simulink model "water_4hopper_open"  (Simulink 8.0)
settings: Solver=ode23  StartTime=0.0  StopTime=30  RelTol=1e-4
values from neighbouring files (symbols this model uses):
  alpha = 30    [SimParam_4VDF.m]
  C_d = 0.703    [SimParam_4VDF.m]
  density = 1000    [SimParam_4VDF.m]
  dTorqueAmp = 0    [SimParam_4VDF.m]
  dTorqueFreq = 0.5    [SimParam_4VDF.m]
  dTorquePhase = 2*pi*rand(1,4)    [SimParam_4VDF.m]
  frame_inertia = diag([Ix,Iy,Iz])    [SimParam_4VDF.m]
  freq = 60    [SimParam_4VDF.m]
  g = 9.81    [SimParam_4VDF.m]
  leg_length = 0.0249    [SimParam_4VDF.m]
  mass = 0.1    [SimParam_4VDF.m]
  S1 = pi*r1^2*0.9185    (= 0.00115422114093)    [SimParam_4VDF.m]
  S2 = pi*r2^2*0.9185    (= 7.21388213081e-05)    [SimParam_4VDF.m]
  tau = 0.005    [SimParam_4VDF.m]
  waveAmp = 0    [SimParam_4VDF.m]
  waveFreq = 0.5    [SimParam_4VDF.m]
undefined symbols (not defined in the file): amp, cw_FL_HL, cw_FR_FL, cw_FR_HR, cw_HR_HL, FL_HL_lag, FR_FL_lag, FR_HR_lag, HR_HL_lag, wavePhase, y_0
libraries: mblibv1 x33
(part 1 of 2)
settings Model: Creator=Metti  LastModifiedBy=nitisht  SimulationMode=rapid-accelerator
settings SolverCC: ZeroCrossControl=DisableAll
settings DataIOCC: SignalLoggingSaveFormat=ModelDataLogs
settings DebuggingCC: FcnCallInpInsideContextMsg=EnableAllAsWarning
settings SimMechanicsCC: VisSampleTime=0.05  AutoFitVis=GROWTOFIT  LastVizWinPosition=[1 41 1600 759]  CamPosition=[-6.20117;3.01965;9.86212;]  CamTarget=[-0.265896;0.0450483;0.16365;]  CamUpVector=[0.0887544;0.966202;-0.242026;]  CamHeight=0.984746  VisBackgroundColor=[0.9;0.9;0.95;]  DefaultBodyColor=[1;0;0;]
settings ConfigurationSet: Description=SimMechanics 2G

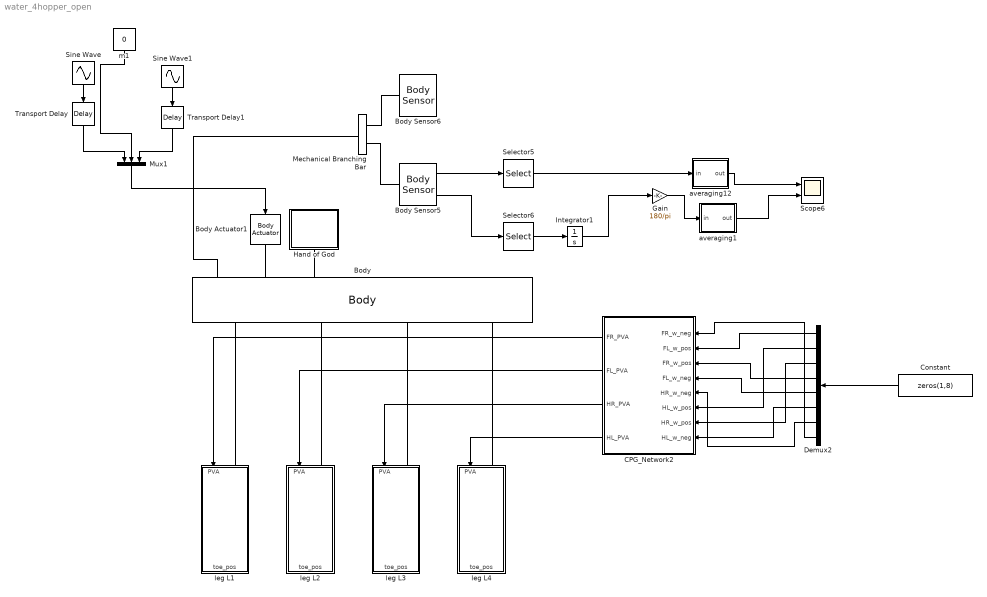
== system water_4hopper_open ==
  Body : mblibv1/Bodies/Body  LConnTagsString=CG|CS10|CS1|CS6|CS7|CS8|CS9  RConnTagsString=CS2|CS3|CS4|CS5  UpdateFromCAD=off  DialogClass=MechanicalBodyBlock  Mass=mass  MassUnits=kg  InertiaUnits=kg*m^2  Inertia=frame_inertia  Shape=Cylinder  ShapeDims=[1 1]  ShapeUnits=m  ShapeUse=false  Density=1  DensityUnits=kg/m^3  DensityUse=false  GraphicsMode=MACHINE_DEFAULT  BodyColorSelMode=MACHINE_DEFAULT  BodyColor=[1 0 0]  AttachedToCS=CG  CG=Left$CG$CG_pos$CS1$CS1$m$[0 0 0]$Euler X-Y-Z$deg$WORLD$true$none  WorkingFrames=Left$CS10$CG_pos$CS1$CS1$m$[0 0 0]$Euler X-Y-Z$deg$WORLD$true$none#Left$CS1$[0 0 0]$Adjoining$Adjoining$m$[0 0 0]$Euler X-Y-Z$deg$WORLD$true$none#Right$CS2$TR_FR$CS1$CS1$m$[0 0 0]$Euler X-Y-Z$deg$WORLD$true$none#Left$CS6$TR_FR$CS1$CS1$m$[0 0 0]$Euler X-Y-Z$deg$WORLD$true$none#Right$CS3$TR_FL$CS1$CS1$m$[0 0 0]$Euler X-Y-Z$deg$WORLD$true$none#Left$CS7$TR_FL$CS1$CS1$m$[0 0 0]$Euler X-Y-Z$deg$WORLD$true$none#Right$CS4$TR_HR$CS1$CS1$m$[0 0 0]$Euler X-Y-Z$deg$WORLD$true$none#Left$CS8$TR_HR$CS1$CS1$m$[0 0 0]$Euler X-Y-Z$deg$WORLD$true$none#Right$CS5$TR_HL$CS1$CS1$m$[0 0 0]$Euler X-Y-Z$deg$WORLD$true$none#Left$CS9$TR_HL$CS1$CS1$m$[0 0 0]$Euler X-Y-Z$deg$WORLD$true$none  CGPos=CG_pos  CGRot=[0 0 0]  CS0Pos=[]  CS0Rot=[]  CS1Pos=[0 0 0]  CS1Rot=[0 0 0]  CS2Pos=TR_FR  CS2Rot=[0 0 0]  CS3Pos=TR_FL  CS3Rot=[0 0 0]  CS4Pos=TR_HR  CS4Rot=[0 0 0]  CS5Pos=TR_HL  CS5Rot=[0 0 0]  CS6Pos=TR_FR  CS6Rot=[0 0 0]  CS7Pos=TR_FL  CS7Rot=[0 0 0]  CS8Pos=TR_HR  CS8Rot=[0 0 0]  CS9Pos=TR_HL  CS9Rot=[0 0 0]  CS10Pos=CG_pos  CS10Rot=[0 0 0]  CS11Pos=[]  CS11Rot=[]  CS12Pos=[]  CS12Rot=[]  CS13Pos=[]  CS13Rot=[]  CS14Pos=[]  CS14Rot=[]  CS15Pos=[]  CS15Rot=[]  CS16Pos=[]  CS16Rot=[]  CS17Pos=[]  CS17Rot=[]  CS18Pos=[]  CS18Rot=[]  CS19Pos=[]  CS19Rot=[]  CS20Pos=[]  CS20Rot=[]
  Body Actuator1 : mblibv1/Sensors &  Actuators/Body Actuator  UpdateFromCAD=off  PhysicalDomain=Mechanical  PortType=blob  ActuationStyle=Force  AngleUnits=deg  ArcVelocityUnits=deg/s  ArcAccelerationUnits=deg/s^2  CoordPositionUnits=m  VelocityUnits=m/s  AccelerationUnits=m/s^2  ForceUnits=N  TorqueUnits=N*m  ActiveIO=on  Width=3  DialogClass=MechanicalActuatorBlock  ReferenceFrame=Absolute (World)  Angle=off  CoordPosition=on  Force=off  Torque=on
  Body Sensor5 : mblibv1/Sensors &  Actuators/Body Sensor  UpdateFromCAD=off  PhysicalDomain=Mechanical  PortType=blob  Muxed=off  Pose=off  Angle=on  AngleUnits=deg  ArcVelocity=on  ArcVelocityUnits=rad/s  ArcAcceleration=off  ArcAccelerationUnits=deg/s^2  CoordPosition=on  CoordPositionUnits=m  Velocity=off  VelocityUnits=m/s  Acceleration=off  AccelerationUnits=m/s^2  Quaternion=on  QuaternionDT=off  QuaternionDDT=off  QuaternionUnits=off  OutputVector=[1]  ActiveIO=on  Width=6  DialogClass=MechanicalSensorBlock  ReferenceFrame=Absolute (World)
  Body Sensor6 : mblibv1/Sensors &  Actuators/Body Sensor  UpdateFromCAD=off  PhysicalDomain=Mechanical  PortType=blob  Muxed=off  Pose=off  Angle=on  AngleUnits=deg  ArcVelocity=on  ArcVelocityUnits=rad/s  ArcAcceleration=off  ArcAccelerationUnits=deg/s^2  CoordPosition=off  CoordPositionUnits=m  Velocity=on  VelocityUnits=m/s  Acceleration=off  AccelerationUnits=m/s^2  Quaternion=on  QuaternionDT=off  QuaternionDDT=off  QuaternionUnits=off  OutputVector=[1]  ActiveIO=on  Width=6  DialogClass=MechanicalSensorBlock  ReferenceFrame=Local (Body CS)
  CPG_Network2 : Subsystem
  Constant : Constant  Value=zeros(1,8)
  Demux2 : Demux  Outputs=8
  Gain : Gain  Gain=180/pi
  Hand of God : Subsystem
  Integrator1 : Integrator
  Mechanical Branching Bar : mblibv1/Utilities/Mechanical Branching Bar  LConnTagsString=_newl0  RConnTagsString=SA0|SA1  UpdateFromCAD=off  DialogClass=MechanicalBranchingBarBlock  NumSAPorts=2
  Mux1 : Mux  Inputs=3
  Scope6 : Scope  NumInputPorts=2
      settings: TimeRange=30  YMin=0.002~-15  YMax=0.01~15  SaveName=ball_position
  Selector5 : Selector  InputPortWidth=3  IndexOptions=Index vector (dialog)  Indices=[2]  OutputSizes=1
  Selector6 : Selector  InputPortWidth=3  IndexOptions=Index vector (dialog)  Indices=[1 3]  OutputSizes=1
  Sine Wave : Sin  Amplitude=dTorqueAmp  Frequency=dTorqueFreq  Phase=dTorquePhase(1)  SampleTime=0
  Sine Wave1 : Sin  Amplitude=dTorqueAmp  Frequency=dTorqueFreq  Phase=dTorquePhase(2)  SampleTime=0
  Transport Delay : TransportDelay  DelayTime=5
  Transport Delay1 : TransportDelay  DelayTime=5
  averaging1 : Subsystem  mask{T_win=2*pi/freq*4, x_init=[ 0, 0]}
      mask prompts: T_win "window (s)"; x_init "Initial condition"
  averaging12 : Subsystem  mask{T_win=2*pi/freq*4, x_init=y_0}
      mask prompts: T_win "window (s)"; x_init "Initial condition"
  leg L1 : Subsystem  mask{wphase=wavePhase(1)}
      mask prompts: wphase "wave phase"
  leg L2 : Subsystem  mask{wphase=wavePhase(2)}
      mask prompts: wphase "wave phase"
  leg L3 : Subsystem  mask{wphase=wavePhase(3)}
      mask prompts: wphase "wave phase"
  leg L4 : Subsystem  mask{wphase=wavePhase(4)}
      mask prompts: wphase "wave phase"
  m1 : Constant  Value=0
  wires:
  Integrator1/1 -> Gain/1
  Body Sensor5/1 -> Selector5/1
  Selector6/1 -> Integrator1/1
  Constant/1 -> Demux2/1
  Demux2/1 -> CPG_Network2/2(FL_w_pos)
  Demux2/5 -> CPG_Network2/4(FL_w_neg)
  Demux2/2 -> CPG_Network2/6(HL_w_pos)
  Demux2/6 -> CPG_Network2/8(HL_w_neg)
  Demux2/3 -> CPG_Network2/7(HR_w_pos)
  Demux2/7 -> CPG_Network2/5(HR_w_neg)
  Demux2/4 -> CPG_Network2/3(FR_w_pos)
  Demux2/8 -> CPG_Network2/1(FR_w_neg)
  CPG_Network2/1(FR_PVA) -> leg L1/1(PVA)
  CPG_Network2/2(FL_PVA) -> leg L2/1(PVA)
  CPG_Network2/3(HR_PVA) -> leg L3/1(PVA)
  CPG_Network2/4(HL_PVA) -> leg L4/1(PVA)
  Gain/1 -> averaging1/1(in)
  Selector5/1 -> averaging12/1(in)
  Body Sensor5/2 -> Selector6/1
  averaging1/1(out) -> Scope6/2
  averaging12/1(out) -> Scope6/1
  Sine Wave/1 -> Transport Delay/1
  Mux1/1 -> Body Actuator1/1
  Transport Delay/1 -> Mux1/1
  Transport Delay1/1 -> Mux1/3
  m1/1 -> Mux1/2
  Sine Wave1/1 -> Transport Delay1/1
  connections:
  Hand of God/RConn1 -- Body/LConn3
  leg L4/LConn1 -- Body/RConn4
  leg L3/LConn1 -- Body/RConn3
  leg L2/LConn1 -- Body/RConn2
  leg L1/LConn1 -- Body/RConn1
  Body/LConn1 -- Mechanical Branching Bar/LConn1
  Mechanical Branching Bar/RConn1 -- Body Sensor6/LConn1
  Mechanical Branching Bar/RConn2 -- Body Sensor5/LConn1
  Body Actuator1/RConn1 -- Body/LConn2

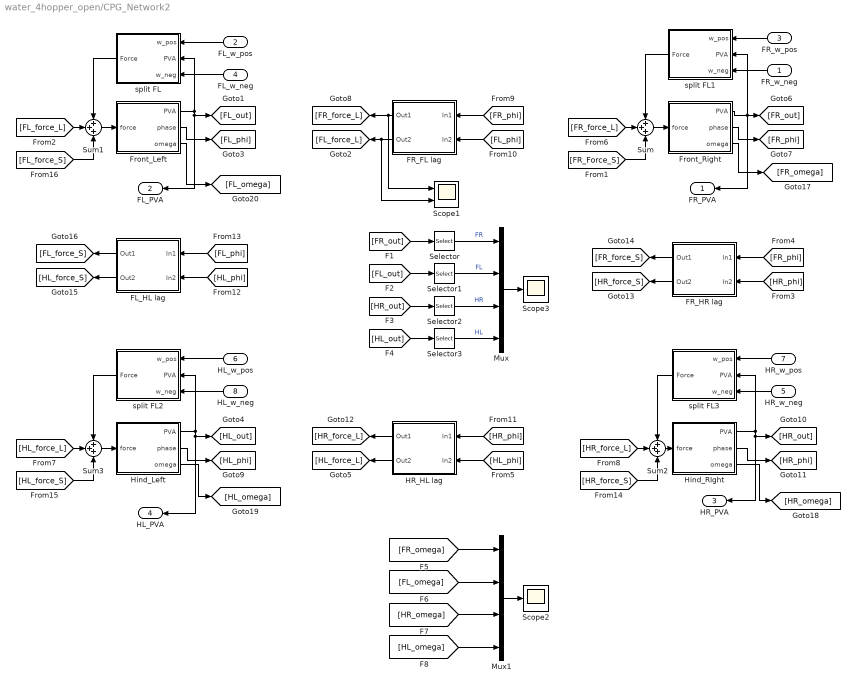
== system water_4hopper_open/CPG_Network2 ==
  FR_w_neg : Inport
  FL_w_pos : Inport  Port=2
  FR_w_pos : Inport  Port=3
  FL_w_neg : Inport  Port=4
  HR_w_neg : Inport  Port=5
  HL_w_pos : Inport  Port=6
  HR_w_pos : Inport  Port=7
  HL_w_neg : Inport  Port=8
  FL_HL lag : Subsystem  mask{d_phase=FL_HL_lag, coupling_weight=cw_FL_HL}
      mask prompts: d_phase "Phase Lag"; coupling_weight "Coupling Weight"
  FR_FL lag : Subsystem  mask{d_phase=FR_FL_lag, coupling_weight=cw_FR_FL}
      mask prompts: d_phase "Phase Lag"; coupling_weight "Coupling Weight"
  FR_HR lag : Subsystem  mask{d_phase=FR_HR_lag, coupling_weight=cw_FR_HR}
      mask prompts: d_phase "Phase Lag"; coupling_weight "Coupling Weight"
  Front_Left : Subsystem  mask{Amp=amp, Offset=0, init_phi=pi}
      mask prompts: Amp "Amplitude"; init_phi "Initial Phase"
  Front_Right : Subsystem  mask{Amp=amp, Offset=0, init_phi=0}
      mask prompts: Amp "Amplitude"; init_phi "Initial Phase"
  HR_HL lag : Subsystem  mask{d_phase=HR_HL_lag, coupling_weight=cw_HR_HL}
      mask prompts: d_phase "Phase Lag"; coupling_weight "Coupling Weight"
  Hind_Left : Subsystem  mask{Amp=amp, Offset=0, init_phi=0}
      mask prompts: Amp "Amplitude"; init_phi "Initial Phase"
  Hind_RIght : Subsystem  mask{Amp=amp, Offset=0, init_phi=pi}
      mask prompts: Amp "Amplitude"; init_phi "Initial Phase"
  Mux : Mux
  Mux1 : Mux
  Scope1 : Scope  NumInputPorts=2
      settings: ShowLegends=on  TimeRange=10  YMin=0~-5  YMax=2~5  SaveName=Output1
  Scope2 : Scope
      settings: ShowLegends=on  TimeRange=20  YMin=68.75  YMax=71.5  SaveName=CPG_omega
  Scope3 : Scope
      settings: ShowLegends=on  TimeRange=10  YMin=-0.025  YMax=0.025  SaveName=Output
  Selector{,1..3} (4 alike) : Selector  InputPortWidth=3  IndexOptions=Index vector (dialog)  Indices=[1]  OutputSizes=1
  Sum{,1..3} (4 alike) : Sum  Inputs=+++
  split FL : Subsystem
  split FL1 : Subsystem
  split FL2 : Subsystem
  split FL3 : Subsystem
  FR_PVA : Outport
  FL_PVA : Outport  Port=2
  HR_PVA : Outport  Port=3
  HL_PVA : Outport  Port=4
  wires:
  Mux/1 -> Scope3/1
  Front_Left/2(phase) -> [FL_phi]
  Front_Right/2(phase) -> [FR_phi]
  [FL_phi] -> FR_FL lag/2(In2)
  [FR_phi] -> FR_FL lag/1(In1)
  FR_FL lag/1(Out1) -> Scope1/1, [FR_force_L]
  FR_FL lag/2(Out2) -> Scope1/2, [FL_force_L]
  Front_Right/1(PVA) -> split FL1/2(PVA), FR_PVA/1, [FR_out]
  [FL_force_L] -> Sum1/2
  Sum1/1 -> Front_Left/1(force)
  Sum/1 -> Front_Right/1(force)
  [FR_force_L] -> Sum/2
  [FL_out] -> Selector1/1
  Selector1/1 -> Mux/2  "FL"
  Selector/1 -> Mux/1  "FR"
  [FR_out] -> Selector/1
  FR_w_pos/1 -> split FL1/1(w_pos)
  FR_w_neg/1 -> split FL1/3(w_neg)
  split FL1/1(Force) -> Sum/1
  FL_w_pos/1 -> split FL/1(w_pos)
  FL_w_neg/1 -> split FL/3(w_neg)
  Front_Left/1(PVA) -> FL_PVA/1, [FL_out], split FL/2(PVA)
  split FL/1(Force) -> Sum1/1
  Hind_Left/2(phase) -> [HL_phi]
  Hind_RIght/2(phase) -> [HR_phi]
  [HL_phi] -> HR_HL lag/2(In2)
  [HR_phi] -> HR_HL lag/1(In1)
  HR_HL lag/1(Out1) -> [HR_force_L]
  HR_HL lag/2(Out2) -> [HL_force_L]
  Hind_RIght/1(PVA) -> HR_PVA/1, [HR_out], split FL3/2(PVA)
  [HL_force_L] -> Sum3/2
  Sum3/1 -> Hind_Left/1(force)
  Sum2/1 -> Hind_RIght/1(force)
  [HR_force_L] -> Sum2/2
  HR_w_pos/1 -> split FL3/1(w_pos)
  HR_w_neg/1 -> split FL3/3(w_neg)
  split FL3/1(Force) -> Sum2/1
  HL_w_pos/1 -> split FL2/1(w_pos)
  HL_w_neg/1 -> split FL2/3(w_neg)
  Hind_Left/1(PVA) -> HL_PVA/1, [HL_out], split FL2/2(PVA)
  split FL2/1(Force) -> Sum3/1
  [HR_phi] -> FR_HR lag/2(In2)
  [FR_phi] -> FR_HR lag/1(In1)
  FR_HR lag/1(Out1) -> [FR_force_S]
  FR_HR lag/2(Out2) -> [HR_force_S]
  [HL_phi] -> FL_HL lag/2(In2)
  [FL_phi] -> FL_HL lag/1(In1)
  FL_HL lag/1(Out1) -> [FL_force_S]
  FL_HL lag/2(Out2) -> [HL_force_S]
  [HL_out] -> Selector3/1
  Selector3/1 -> Mux/4  "HL"
  Selector2/1 -> Mux/3  "HR"
  [HR_out] -> Selector2/1
  [FR_Force_S] -> Sum/3
  [HR_force_S] -> Sum2/3
  [HL_force_S] -> Sum3/3
  [FL_force_S] -> Sum1/3
  Front_Right/3(omega) -> [FR_omega]
  Hind_RIght/3(omega) -> [HR_omega]
  Hind_Left/3(omega) -> [HL_omega]
  Front_Left/3(omega) -> [FL_omega]
  Mux1/1 -> Scope2/1
  [FR_omega] -> Mux1/1
  [HL_omega] -> Mux1/4
  [HR_omega] -> Mux1/3
  [FL_omega] -> Mux1/2

== system water_4hopper_open/Hand of God ==
  Custom Joint : mblibv1/Joints/Custom Joint  LConnTagsString=__newl0|SA1  RConnTagsString=__newr0  UpdateFromCAD=off  NumSAPorts=1  CutJoint=off  MarkAsCut=off  Primitives=prismatic  PrimitiveProps=P1$World$[0 1 0]$Prismatic#R1$World$[1 0 0]$Revolute#R2$World$[0 0 1]$Revolute  DialogClass=JointBlock  R1Axis=[1 0 0]  R2Axis=[0 0 1]  R3Axis=[]  P1Axis=[0 1 0]  P2Axis=[]  P3Axis=[]  SAxis=[]
  Ground : mblibv1/Bodies/Ground  UpdateFromCAD=off  LeftPortType=env  RightPortType=workingframe  PhysicalDomain=Mechanical  DialogClass=GroundBlock  CoordPosition=[0 0 0]  CoordPositionUnits=m  StateVectorMgrId=1  MachineId=[2 0]  ShowEnvPort=on
  Joint Initial Condition : mblibv1/Sensors &  Actuators/Joint Initial Condition  UpdateFromCAD=off  LeftPortType=blob  RightPortType=blob  PhysicalDomain=mechanical  DialogClass=InitialConditionBlock  InitialConditions=P1$true$y_0$m$deg$0$m/s$deg/s#P2$false$0$m$deg$0$m/s$deg/s#P3$false$0$m$deg$0$m/s$deg/s#R1$true$0$m$deg$0$m/s$deg/s#R2$true$0$m$deg$0$m/s$deg/s#R3$false$10$m$deg$0$m/s$deg/s#S$false$0$m$deg$0$m/s$deg/s  P1PIC=y_0  P1VIC=0  P2PIC=0  P2VIC=0  P3PIC=0  P3VIC=0  R1PIC=0  R1VIC=0  R2PIC=0  R2VIC=0  R3PIC=0  R3VIC=0  SPIC=0  SVIC=0
  Joint Sensor : mblibv1/Sensors &  Actuators/Joint Sensor  UpdateFromCAD=off  PhysicalDomain=Mechanical  PortType=blob  Muxed=on  Pose=off  Angle=on  AngleUnits=deg  ArcVelocity=off  ArcVelocityUnits=deg/s  ArcAcceleration=off  ArcAccelerationUnits=deg/s^2  CoordPosition=on  CoordPositionUnits=m  Velocity=off  VelocityUnits=m/s  Acceleration=off  AccelerationUnits=m/s^2  Quaternion=on  QuaternionDT=off  QuaternionDDT=off  QuaternionUnits=off  OutputVector=[1]  ActiveIO=on  Width=1  DialogClass=MechanicalSensorBlock  Primitive=P1  Force=off  ForceUnits=N  Torque=off  TorqueUnits=N*m  ReferenceFrame=Absolute (World)  ReactionSensedSide=Base  ReactionReferenceFrame=Absolute (World)  ReactionForce=off  ReactionForceUnits=N  ReactionMoment=off  ReactionMomentUnits=N*m
  Joint Sensor1 : mblibv1/Sensors &  Actuators/Joint Sensor  UpdateFromCAD=off  PhysicalDomain=Mechanical  PortType=blob  Muxed=on  Pose=off  Angle=on  AngleUnits=deg  ArcVelocity=off  ArcVelocityUnits=deg/s  ArcAcceleration=off  ArcAccelerationUnits=deg/s^2  CoordPosition=off  CoordPositionUnits=m  Velocity=on  VelocityUnits=m/s  Acceleration=off  AccelerationUnits=m/s^2  Quaternion=on  QuaternionDT=off  QuaternionDDT=off  QuaternionUnits=off  OutputVector=[1]  ActiveIO=on  Width=1  DialogClass=MechanicalSensorBlock  Primitive=R1  Force=off  ForceUnits=N  Torque=off  TorqueUnits=N*m  ReferenceFrame=Absolute (World)  ReactionSensedSide=Base  ReactionReferenceFrame=Absolute (World)  ReactionForce=off  ReactionForceUnits=N  ReactionMoment=off  ReactionMomentUnits=N*m
  Joint Sensor2 : mblibv1/Sensors &  Actuators/Joint Sensor  UpdateFromCAD=off  PhysicalDomain=Mechanical  PortType=blob  Muxed=off  Pose=off  Angle=on  AngleUnits=deg  ArcVelocity=off  ArcVelocityUnits=deg/s  ArcAcceleration=off  ArcAccelerationUnits=deg/s^2  CoordPosition=on  CoordPositionUnits=m  Velocity=off  VelocityUnits=m/s  Acceleration=off  AccelerationUnits=m/s^2  Quaternion=on  QuaternionDT=off  QuaternionDDT=off  QuaternionUnits=off  OutputVector=[1]  ActiveIO=on  Width=1  DialogClass=MechanicalSensorBlock  Primitive=R2  Force=off  ForceUnits=N  Torque=off  TorqueUnits=N*m  ReferenceFrame=Absolute (World)  ReactionSensedSide=Base  ReactionReferenceFrame=Absolute (World)  ReactionForce=off  ReactionForceUnits=N  ReactionMoment=off  ReactionMomentUnits=N*m
  Machine Environment : mblibv1/Bodies/Machine Environment  PortType=env  PhysicalDomain=Mechanical  DialogTemplateClass=MECH.MachineEnvironment  SyncWhenCopied=off  Gravity=[0 -g 0]  GravityUnits=m/s^2  GravityAsSignal=off  Dimensionality=Auto-detect  AnalysisType=Forward dynamics  LinearAssemblyTolerance=1e-3  LinearAssemblyToleranceUnits=m  AngularAssemblyTolerance=1e-3  AngularAssemblyToleranceUnits=rad  ConstraintSolverType=Stabilizing  ConstraintRelTolerance=1e-4  ConstraintAbsTolerance=1e-4  UseRobustSingularityHandling=off  RedundancyAnalysisToleranceType=Automatically select tolerance  RedundancyAnalysisTolerance=1e-14  StatePerturbationType=Fixed  PerturbationSize=1e-5  VisualizeMachine=on  BodyVisualizationType=Use model default body geometries  BodyColorSelMode=Use model default  DefaultBodyColor=[1 0 0]
  Mechanical Branching Bar : mblibv1/Utilities/Mechanical Branching Bar  LConnTagsString=_newl0  RConnTagsString=__newr0|SA2|SA3|SA4  UpdateFromCAD=off  DialogClass=MechanicalBranchingBarBlock  NumSAPorts=4
  Scope : Scope  NumInputPorts=3
      settings: TimeRange=5  YMin=-0.01~-0.001~-6  YMax=0.02~0.0004~1  SaveName=mass_data
  Conn1 : PMIOPort  Port=1  Side=Right
  wires:
  Joint Sensor/1 -> Scope/1
  Joint Sensor1/1 -> Scope/2
  Joint Sensor2/1 -> Scope/3
  connections:
  Conn1/RConn1 -- Custom Joint/RConn1
  Joint Sensor1/LConn1 -- Mechanical Branching Bar/RConn3
  Ground/RConn1 -- Custom Joint/LConn1
  Machine Environment/RConn1 -- Ground/LConn1
  Joint Initial Condition/RConn1 -- Mechanical Branching Bar/RConn1
  Joint Sensor/LConn1 -- Mechanical Branching Bar/RConn2
  Custom Joint/LConn2 -- Mechanical Branching Bar/LConn1
  Joint Sensor2/LConn1 -- Mechanical Branching Bar/RConn4

== system water_4hopper_open/averaging1 ==
  in : Inport
  Constant1 : Constant  Value=x_init
  Gain : Gain  Gain=1/T_win
  Integrator1 : Integrator
  Sum : Sum  Inputs=+-|
  Sum1 : Sum  Inputs=-+|
  Sum3 : Sum  Inputs=++|
  Transport Delay : TransportDelay  DelayTime=T_win
  out : Outport
  wires:
  in/1 -> Sum1/2
  Gain/1 -> Sum3/2
  Constant1/1 -> Sum3/1, Sum1/1
  Sum1/1 -> Integrator1/1
  Transport Delay/1 -> Sum/2
  Integrator1/1 -> Sum/1, Transport Delay/1
  Sum3/1 -> out/1
  Sum/1 -> Gain/1

== system water_4hopper_open/averaging12 ==
  in : Inport
  Constant1 : Constant  Value=x_init
  Gain : Gain  Gain=1/T_win
  Integrator1 : Integrator
  Sum : Sum  Inputs=+-|
  Sum1 : Sum  Inputs=-+|
  Sum3 : Sum  Inputs=++|
  Transport Delay : TransportDelay  DelayTime=T_win
  out : Outport
  wires:
  in/1 -> Sum1/2
  Gain/1 -> Sum3/2
  Constant1/1 -> Sum3/1, Sum1/1
  Sum1/1 -> Integrator1/1
  Transport Delay/1 -> Sum/2
  Integrator1/1 -> Sum/1, Transport Delay/1
  Sum3/1 -> out/1
  Sum/1 -> Gain/1

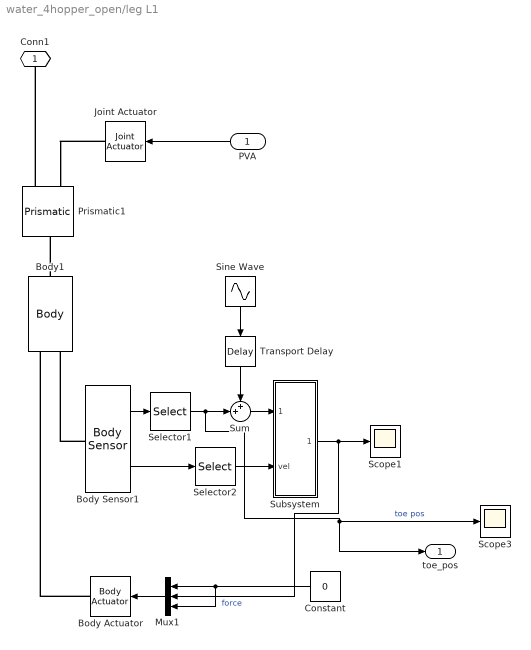
== system water_4hopper_open/leg L1 ==
  PVA : Inport
  Body Actuator : mblibv1/Sensors &  Actuators/Body Actuator  UpdateFromCAD=off  PhysicalDomain=Mechanical  PortType=blob  ActuationStyle=Force  AngleUnits=deg  ArcVelocityUnits=deg/s  ArcAccelerationUnits=deg/s^2  CoordPositionUnits=m  VelocityUnits=m/s  AccelerationUnits=m/s^2  ForceUnits=N  TorqueUnits=N*m  ActiveIO=on  Width=3  DialogClass=MechanicalActuatorBlock  ReferenceFrame=Local (Body CS)  Angle=off  CoordPosition=on  Force=on  Torque=off
  Body Sensor1 : mblibv1/Sensors &  Actuators/Body Sensor  UpdateFromCAD=off  PhysicalDomain=Mechanical  PortType=blob  Muxed=off  Pose=off  Angle=on  AngleUnits=deg  ArcVelocity=off  ArcVelocityUnits=deg/s  ArcAcceleration=off  ArcAccelerationUnits=deg/s^2  CoordPosition=on  CoordPositionUnits=m  Velocity=on  VelocityUnits=m/s  Acceleration=off  AccelerationUnits=m/s^2  Quaternion=on  QuaternionDT=off  QuaternionDDT=off  QuaternionUnits=off  OutputVector=[1]  ActiveIO=on  Width=6  DialogClass=MechanicalSensorBlock  ReferenceFrame=Absolute (World)
  Body1 : mblibv1/Bodies/Body  LConnTagsString=CS1  RConnTagsString=CS2|CS3  UpdateFromCAD=off  DialogClass=MechanicalBodyBlock  Mass=0  MassUnits=kg  InertiaUnits=kg*m^2  Inertia=zeros(3)  Shape=Cylinder  ShapeDims=[1 1]  ShapeUnits=m  ShapeUse=false  Density=1  DensityUnits=kg/m^3  DensityUse=false  GraphicsMode=MACHINE_DEFAULT  BodyColorSelMode=MACHINE_DEFAULT  BodyColor=[1 0 0]  AttachedToCS=CG  CG=Left$CG$[0 -leg_length 0]$CS1$CS1$m$[0 0 0]$Euler X-Y-Z$deg$WORLD$false$none  WorkingFrames=Left$CS1$[0 0 0]$Adjoining$Adjoining$m$[0 0 0]$Euler X-Y-Z$deg$WORLD$true$none#Right$CS2$[0 -leg_length 0]$CS1$CS1$m$[0 0 0]$Euler X-Y-Z$deg$WORLD$true$none#Right$CS3$[0 -leg_length 0]$CS1$CS1$m$[0 0 0]$Euler X-Y-Z$deg$WORLD$true$none  CGPos=[0 -leg_length 0]  CGRot=[0 0 0]  CS0Pos=[]  CS0Rot=[]  CS1Pos=[0 0 0]  CS1Rot=[0 0 0]  CS2Pos=[0 -leg_length 0]  CS2Rot=[0 0 0]  CS3Pos=[0 -leg_length 0]  CS3Rot=[0 0 0]  CS4Pos=[]  CS4Rot=[]  CS5Pos=[]  CS5Rot=[]  CS6Pos=[]  CS6Rot=[]  CS7Pos=[]  CS7Rot=[]  CS8Pos=[]  CS8Rot=[]  CS9Pos=[]  CS9Rot=[]  CS10Pos=[]  CS10Rot=[]  CS11Pos=[]  CS11Rot=[]  CS12Pos=[]  CS12Rot=[]  CS13Pos=[]  CS13Rot=[]  CS14Pos=[]  CS14Rot=[]  CS15Pos=[]  CS15Rot=[]  CS16Pos=[]  CS16Rot=[]  CS17Pos=[]  CS17Rot=[]  CS18Pos=[]  CS18Rot=[]  CS19Pos=[]  CS19Rot=[]  CS20Pos=[]  CS20Rot=[]
  Constant : Constant  Value=0
  Joint Actuator : mblibv1/Sensors &  Actuators/Joint Actuator  UpdateFromCAD=off  PhysicalDomain=Mechanical  PortType=blob  ActuationStyle=Motion  AngleUnits=deg  ArcVelocityUnits=deg/s  ArcAccelerationUnits=deg/s^2  CoordPositionUnits=m  VelocityUnits=m/s  AccelerationUnits=m/s^2  ForceUnits=N  TorqueUnits=N*m  ActiveIO=on  Width=3  DialogClass=MechanicalActuatorBlock  Primitive=P1  ReferenceFrame=Absolute (World)
  Mux1 : Mux  Inputs=3
  Prismatic1 : mblibv1/Joints/Prismatic  LConnTagsString=__newl0|SA1  RConnTagsString=__newr0  UpdateFromCAD=off  NumSAPorts=1  CutJoint=off  MarkAsCut=off  Primitives=prismatic  PrimitiveProps=P1$World$[0 1 0]$prismatic  DialogClass=JointBlock  P1Axis=[0 1 0]
  Scope1 : Scope
      settings: SaveName=force_L
  Scope3 : Scope
      settings: SaveName=toe_position_L
  Selector1 : Selector  InputPortWidth=3  IndexOptions=Index vector (dialog)  Indices=[2]  OutputSizes=1
  Selector2 : Selector  InputPortWidth=3  IndexOptions=Index vector (dialog)  Indices=[2]  OutputSizes=1
  Sine Wave : Sin  Amplitude=waveAmp  Frequency=waveFreq  Phase=wphase  SampleTime=0
  Subsystem : Subsystem
  Sum : Sum  Inputs=++|
  Transport Delay : TransportDelay  DelayTime=5
  Conn1 : PMIOPort  Port=1  Side=Left
  toe_pos : Outport
  wires:
  Body Sensor1/2 -> Selector2/1
  Selector1/1 -> Sum/2, Scope3/1, toe_pos/1  "toe pos"
  Selector2/1 -> Subsystem/2(vel)
  Subsystem/1(force) -> Scope1/1, Mux1/2  "force"
  Mux1/1 -> Body Actuator/1
  Constant/1 -> Mux1/1, Mux1/3
  PVA/1 -> Joint Actuator/1
  Body Sensor1/1 -> Selector1/1
  Sine Wave/1 -> Transport Delay/1
  Sum/1 -> Subsystem/1(pos)
  Transport Delay/1 -> Sum/1
  connections:
  Body1/LConn1 -- Prismatic1/RConn1
  Body Actuator/RConn1 -- Body1/RConn1
  Body Sensor1/LConn1 -- Body1/RConn2
  Prismatic1/LConn1 -- Conn1/RConn1
  Joint Actuator/RConn1 -- Prismatic1/LConn2

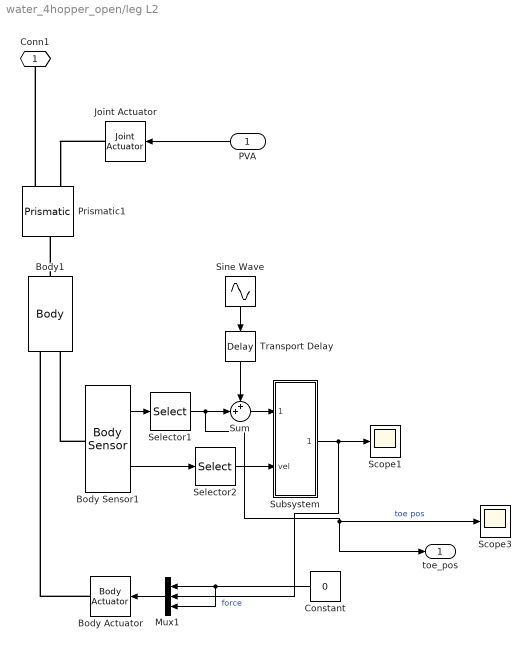
== system water_4hopper_open/leg L2 ==
  PVA : Inport
  Body Actuator : mblibv1/Sensors &  Actuators/Body Actuator  UpdateFromCAD=off  PhysicalDomain=Mechanical  PortType=blob  ActuationStyle=Force  AngleUnits=deg  ArcVelocityUnits=deg/s  ArcAccelerationUnits=deg/s^2  CoordPositionUnits=m  VelocityUnits=m/s  AccelerationUnits=m/s^2  ForceUnits=N  TorqueUnits=N*m  ActiveIO=on  Width=3  DialogClass=MechanicalActuatorBlock  ReferenceFrame=Local (Body CS)  Angle=off  CoordPosition=on  Force=on  Torque=off
  Body Sensor1 : mblibv1/Sensors &  Actuators/Body Sensor  UpdateFromCAD=off  PhysicalDomain=Mechanical  PortType=blob  Muxed=off  Pose=off  Angle=on  AngleUnits=deg  ArcVelocity=off  ArcVelocityUnits=deg/s  ArcAcceleration=off  ArcAccelerationUnits=deg/s^2  CoordPosition=on  CoordPositionUnits=m  Velocity=on  VelocityUnits=m/s  Acceleration=off  AccelerationUnits=m/s^2  Quaternion=on  QuaternionDT=off  QuaternionDDT=off  QuaternionUnits=off  OutputVector=[1]  ActiveIO=on  Width=6  DialogClass=MechanicalSensorBlock  ReferenceFrame=Absolute (World)
  Body1 : mblibv1/Bodies/Body  LConnTagsString=CS1  RConnTagsString=CS2|CS3  UpdateFromCAD=off  DialogClass=MechanicalBodyBlock  Mass=0  MassUnits=kg  InertiaUnits=kg*m^2  Inertia=zeros(3)  Shape=Cylinder  ShapeDims=[1 1]  ShapeUnits=m  ShapeUse=false  Density=1  DensityUnits=kg/m^3  DensityUse=false  GraphicsMode=MACHINE_DEFAULT  BodyColorSelMode=MACHINE_DEFAULT  BodyColor=[1 0 0]  AttachedToCS=CG  CG=Left$CG$[0 -leg_length 0]$CS1$CS1$m$[0 0 0]$Euler X-Y-Z$deg$WORLD$false$none  WorkingFrames=Left$CS1$[0 0 0]$Adjoining$Adjoining$m$[0 0 0]$Euler X-Y-Z$deg$WORLD$true$none#Right$CS2$[0 -leg_length 0]$CS1$CS1$m$[0 0 0]$Euler X-Y-Z$deg$WORLD$true$none#Right$CS3$[0 -leg_length 0]$CS1$CS1$m$[0 0 0]$Euler X-Y-Z$deg$WORLD$true$none  CGPos=[0 -leg_length 0]  CGRot=[0 0 0]  CS0Pos=[]  CS0Rot=[]  CS1Pos=[0 0 0]  CS1Rot=[0 0 0]  CS2Pos=[0 -leg_length 0]  CS2Rot=[0 0 0]  CS3Pos=[0 -leg_length 0]  CS3Rot=[0 0 0]  CS4Pos=[]  CS4Rot=[]  CS5Pos=[]  CS5Rot=[]  CS6Pos=[]  CS6Rot=[]  CS7Pos=[]  CS7Rot=[]  CS8Pos=[]  CS8Rot=[]  CS9Pos=[]  CS9Rot=[]  CS10Pos=[]  CS10Rot=[]  CS11Pos=[]  CS11Rot=[]  CS12Pos=[]  CS12Rot=[]  CS13Pos=[]  CS13Rot=[]  CS14Pos=[]  CS14Rot=[]  CS15Pos=[]  CS15Rot=[]  CS16Pos=[]  CS16Rot=[]  CS17Pos=[]  CS17Rot=[]  CS18Pos=[]  CS18Rot=[]  CS19Pos=[]  CS19Rot=[]  CS20Pos=[]  CS20Rot=[]
  Constant : Constant  Value=0
  Joint Actuator : mblibv1/Sensors &  Actuators/Joint Actuator  UpdateFromCAD=off  PhysicalDomain=Mechanical  PortType=blob  ActuationStyle=Motion  AngleUnits=deg  ArcVelocityUnits=deg/s  ArcAccelerationUnits=deg/s^2  CoordPositionUnits=m  VelocityUnits=m/s  AccelerationUnits=m/s^2  ForceUnits=N  TorqueUnits=N*m  ActiveIO=on  Width=3  DialogClass=MechanicalActuatorBlock  Primitive=P1  ReferenceFrame=Absolute (World)
  Mux1 : Mux  Inputs=3
  Prismatic1 : mblibv1/Joints/Prismatic  LConnTagsString=__newl0|SA1  RConnTagsString=__newr0  UpdateFromCAD=off  NumSAPorts=1  CutJoint=off  MarkAsCut=off  Primitives=prismatic  PrimitiveProps=P1$World$[0 1 0]$prismatic  DialogClass=JointBlock  P1Axis=[0 1 0]
  Scope1 : Scope
      settings: SaveName=force_L
  Scope3 : Scope
      settings: SaveName=toe_position_L
  Selector1 : Selector  InputPortWidth=3  IndexOptions=Index vector (dialog)  Indices=[2]  OutputSizes=1
  Selector2 : Selector  InputPortWidth=3  IndexOptions=Index vector (dialog)  Indices=[2]  OutputSizes=1
  Sine Wave : Sin  Amplitude=waveAmp  Frequency=waveFreq  Phase=wphase  SampleTime=0
  Subsystem : Subsystem
  Sum : Sum  Inputs=++|
  Transport Delay : TransportDelay  DelayTime=5
  Conn1 : PMIOPort  Port=1  Side=Left
  toe_pos : Outport
  wires:
  Body Sensor1/2 -> Selector2/1
  Selector1/1 -> Sum/2, Scope3/1, toe_pos/1  "toe pos"
  Selector2/1 -> Subsystem/2(vel)
  Subsystem/1(force) -> Scope1/1, Mux1/2  "force"
  Mux1/1 -> Body Actuator/1
  Constant/1 -> Mux1/1, Mux1/3
  PVA/1 -> Joint Actuator/1
  Body Sensor1/1 -> Selector1/1
  Sine Wave/1 -> Transport Delay/1
  Sum/1 -> Subsystem/1(pos)
  Transport Delay/1 -> Sum/1
  connections:
  Body1/LConn1 -- Prismatic1/RConn1
  Body Actuator/RConn1 -- Body1/RConn1
  Body Sensor1/LConn1 -- Body1/RConn2
  Prismatic1/LConn1 -- Conn1/RConn1
  Joint Actuator/RConn1 -- Prismatic1/LConn2

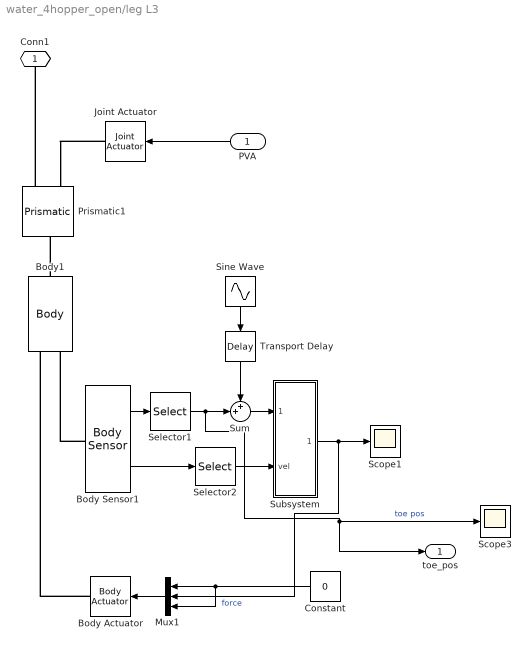
== system water_4hopper_open/leg L3 ==
  PVA : Inport
  Body Actuator : mblibv1/Sensors &  Actuators/Body Actuator  UpdateFromCAD=off  PhysicalDomain=Mechanical  PortType=blob  ActuationStyle=Force  AngleUnits=deg  ArcVelocityUnits=deg/s  ArcAccelerationUnits=deg/s^2  CoordPositionUnits=m  VelocityUnits=m/s  AccelerationUnits=m/s^2  ForceUnits=N  TorqueUnits=N*m  ActiveIO=on  Width=3  DialogClass=MechanicalActuatorBlock  ReferenceFrame=Local (Body CS)  Angle=off  CoordPosition=on  Force=on  Torque=off
  Body Sensor1 : mblibv1/Sensors &  Actuators/Body Sensor  UpdateFromCAD=off  PhysicalDomain=Mechanical  PortType=blob  Muxed=off  Pose=off  Angle=on  AngleUnits=deg  ArcVelocity=off  ArcVelocityUnits=deg/s  ArcAcceleration=off  ArcAccelerationUnits=deg/s^2  CoordPosition=on  CoordPositionUnits=m  Velocity=on  VelocityUnits=m/s  Acceleration=off  AccelerationUnits=m/s^2  Quaternion=on  QuaternionDT=off  QuaternionDDT=off  QuaternionUnits=off  OutputVector=[1]  ActiveIO=on  Width=6  DialogClass=MechanicalSensorBlock  ReferenceFrame=Absolute (World)
  Body1 : mblibv1/Bodies/Body  LConnTagsString=CS1  RConnTagsString=CS2|CS3  UpdateFromCAD=off  DialogClass=MechanicalBodyBlock  Mass=0  MassUnits=kg  InertiaUnits=kg*m^2  Inertia=zeros(3)  Shape=Cylinder  ShapeDims=[1 1]  ShapeUnits=m  ShapeUse=false  Density=1  DensityUnits=kg/m^3  DensityUse=false  GraphicsMode=MACHINE_DEFAULT  BodyColorSelMode=MACHINE_DEFAULT  BodyColor=[1 0 0]  AttachedToCS=CG  CG=Left$CG$[0 -leg_length 0]$CS1$CS1$m$[0 0 0]$Euler X-Y-Z$deg$WORLD$false$none  WorkingFrames=Left$CS1$[0 0 0]$Adjoining$Adjoining$m$[0 0 0]$Euler X-Y-Z$deg$WORLD$true$none#Right$CS2$[0 -leg_length 0]$CS1$CS1$m$[0 0 0]$Euler X-Y-Z$deg$WORLD$true$none#Right$CS3$[0 -leg_length 0]$CS1$CS1$m$[0 0 0]$Euler X-Y-Z$deg$WORLD$true$none  CGPos=[0 -leg_length 0]  CGRot=[0 0 0]  CS0Pos=[]  CS0Rot=[]  CS1Pos=[0 0 0]  CS1Rot=[0 0 0]  CS2Pos=[0 -leg_length 0]  CS2Rot=[0 0 0]  CS3Pos=[0 -leg_length 0]  CS3Rot=[0 0 0]  CS4Pos=[]  CS4Rot=[]  CS5Pos=[]  CS5Rot=[]  CS6Pos=[]  CS6Rot=[]  CS7Pos=[]  CS7Rot=[]  CS8Pos=[]  CS8Rot=[]  CS9Pos=[]  CS9Rot=[]  CS10Pos=[]  CS10Rot=[]  CS11Pos=[]  CS11Rot=[]  CS12Pos=[]  CS12Rot=[]  CS13Pos=[]  CS13Rot=[]  CS14Pos=[]  CS14Rot=[]  CS15Pos=[]  CS15Rot=[]  CS16Pos=[]  CS16Rot=[]  CS17Pos=[]  CS17Rot=[]  CS18Pos=[]  CS18Rot=[]  CS19Pos=[]  CS19Rot=[]  CS20Pos=[]  CS20Rot=[]
  Constant : Constant  Value=0
  Joint Actuator : mblibv1/Sensors &  Actuators/Joint Actuator  UpdateFromCAD=off  PhysicalDomain=Mechanical  PortType=blob  ActuationStyle=Motion  AngleUnits=deg  ArcVelocityUnits=deg/s  ArcAccelerationUnits=deg/s^2  CoordPositionUnits=m  VelocityUnits=m/s  AccelerationUnits=m/s^2  ForceUnits=N  TorqueUnits=N*m  ActiveIO=on  Width=3  DialogClass=MechanicalActuatorBlock  Primitive=P1  ReferenceFrame=Absolute (World)
  Mux1 : Mux  Inputs=3
  Prismatic1 : mblibv1/Joints/Prismatic  LConnTagsString=__newl0|SA1  RConnTagsString=__newr0  UpdateFromCAD=off  NumSAPorts=1  CutJoint=off  MarkAsCut=off  Primitives=prismatic  PrimitiveProps=P1$World$[0 1 0]$prismatic  DialogClass=JointBlock  P1Axis=[0 1 0]
  Scope1 : Scope
      settings: SaveName=force_L
  Scope3 : Scope
      settings: SaveName=toe_position_L
  Selector1 : Selector  InputPortWidth=3  IndexOptions=Index vector (dialog)  Indices=[2]  OutputSizes=1
  Selector2 : Selector  InputPortWidth=3  IndexOptions=Index vector (dialog)  Indices=[2]  OutputSizes=1
  Sine Wave : Sin  Amplitude=waveAmp  Frequency=waveFreq  Phase=wphase  SampleTime=0
  Subsystem : Subsystem
  Sum : Sum  Inputs=++|
  Transport Delay : TransportDelay  DelayTime=5
  Conn1 : PMIOPort  Port=1  Side=Left
  toe_pos : Outport
  wires:
  Body Sensor1/2 -> Selector2/1
  Selector1/1 -> Sum/2, Scope3/1, toe_pos/1  "toe pos"
  Selector2/1 -> Subsystem/2(vel)
  Subsystem/1(force) -> Scope1/1, Mux1/2  "force"
  Mux1/1 -> Body Actuator/1
  Constant/1 -> Mux1/1, Mux1/3
  PVA/1 -> Joint Actuator/1
  Body Sensor1/1 -> Selector1/1
  Sine Wave/1 -> Transport Delay/1
  Sum/1 -> Subsystem/1(pos)
  Transport Delay/1 -> Sum/1
  connections:
  Body1/LConn1 -- Prismatic1/RConn1
  Body Actuator/RConn1 -- Body1/RConn1
  Body Sensor1/LConn1 -- Body1/RConn2
  Prismatic1/LConn1 -- Conn1/RConn1
  Joint Actuator/RConn1 -- Prismatic1/LConn2

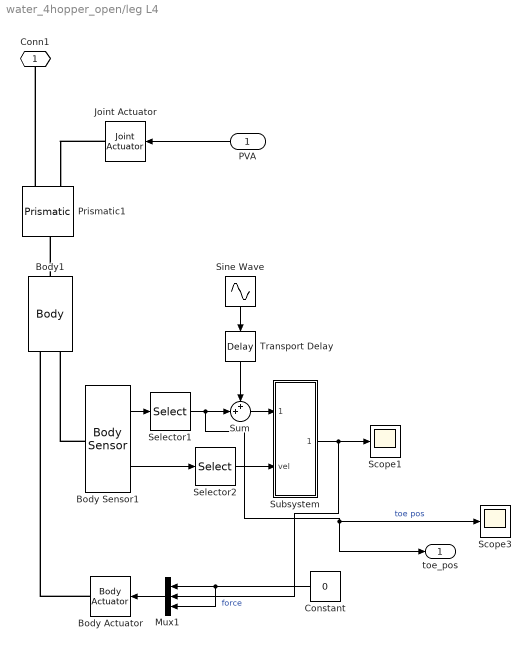
== system water_4hopper_open/leg L4 ==
  PVA : Inport
  Body Actuator : mblibv1/Sensors &  Actuators/Body Actuator  UpdateFromCAD=off  PhysicalDomain=Mechanical  PortType=blob  ActuationStyle=Force  AngleUnits=deg  ArcVelocityUnits=deg/s  ArcAccelerationUnits=deg/s^2  CoordPositionUnits=m  VelocityUnits=m/s  AccelerationUnits=m/s^2  ForceUnits=N  TorqueUnits=N*m  ActiveIO=on  Width=3  DialogClass=MechanicalActuatorBlock  ReferenceFrame=Local (Body CS)  Angle=off  CoordPosition=on  Force=on  Torque=off
  Body Sensor1 : mblibv1/Sensors &  Actuators/Body Sensor  UpdateFromCAD=off  PhysicalDomain=Mechanical  PortType=blob  Muxed=off  Pose=off  Angle=on  AngleUnits=deg  ArcVelocity=off  ArcVelocityUnits=deg/s  ArcAcceleration=off  ArcAccelerationUnits=deg/s^2  CoordPosition=on  CoordPositionUnits=m  Velocity=on  VelocityUnits=m/s  Acceleration=off  AccelerationUnits=m/s^2  Quaternion=on  QuaternionDT=off  QuaternionDDT=off  QuaternionUnits=off  OutputVector=[1]  ActiveIO=on  Width=6  DialogClass=MechanicalSensorBlock  ReferenceFrame=Absolute (World)
  Body1 : mblibv1/Bodies/Body  LConnTagsString=CS1  RConnTagsString=CS2|CS3  UpdateFromCAD=off  DialogClass=MechanicalBodyBlock  Mass=0  MassUnits=kg  InertiaUnits=kg*m^2  Inertia=zeros(3)  Shape=Cylinder  ShapeDims=[1 1]  ShapeUnits=m  ShapeUse=false  Density=1  DensityUnits=kg/m^3  DensityUse=false  GraphicsMode=MACHINE_DEFAULT  BodyColorSelMode=MACHINE_DEFAULT  BodyColor=[1 0 0]  AttachedToCS=CG  CG=Left$CG$[0 -leg_length 0]$CS1$CS1$m$[0 0 0]$Euler X-Y-Z$deg$WORLD$false$none  WorkingFrames=Left$CS1$[0 0 0]$Adjoining$Adjoining$m$[0 0 0]$Euler X-Y-Z$deg$WORLD$true$none#Right$CS2$[0 -leg_length 0]$CS1$CS1$m$[0 0 0]$Euler X-Y-Z$deg$WORLD$true$none#Right$CS3$[0 -leg_length 0]$CS1$CS1$m$[0 0 0]$Euler X-Y-Z$deg$WORLD$true$none  CGPos=[0 -leg_length 0]  CGRot=[0 0 0]  CS0Pos=[]  CS0Rot=[]  CS1Pos=[0 0 0]  CS1Rot=[0 0 0]  CS2Pos=[0 -leg_length 0]  CS2Rot=[0 0 0]  CS3Pos=[0 -leg_length 0]  CS3Rot=[0 0 0]  CS4Pos=[]  CS4Rot=[]  CS5Pos=[]  CS5Rot=[]  CS6Pos=[]  CS6Rot=[]  CS7Pos=[]  CS7Rot=[]  CS8Pos=[]  CS8Rot=[]  CS9Pos=[]  CS9Rot=[]  CS10Pos=[]  CS10Rot=[]  CS11Pos=[]  CS11Rot=[]  CS12Pos=[]  CS12Rot=[]  CS13Pos=[]  CS13Rot=[]  CS14Pos=[]  CS14Rot=[]  CS15Pos=[]  CS15Rot=[]  CS16Pos=[]  CS16Rot=[]  CS17Pos=[]  CS17Rot=[]  CS18Pos=[]  CS18Rot=[]  CS19Pos=[]  CS19Rot=[]  CS20Pos=[]  CS20Rot=[]
  Constant : Constant  Value=0
  Joint Actuator : mblibv1/Sensors &  Actuators/Joint Actuator  UpdateFromCAD=off  PhysicalDomain=Mechanical  PortType=blob  ActuationStyle=Motion  AngleUnits=deg  ArcVelocityUnits=deg/s  ArcAccelerationUnits=deg/s^2  CoordPositionUnits=m  VelocityUnits=m/s  AccelerationUnits=m/s^2  ForceUnits=N  TorqueUnits=N*m  ActiveIO=on  Width=3  DialogClass=MechanicalActuatorBlock  Primitive=P1  ReferenceFrame=Absolute (World)
  Mux1 : Mux  Inputs=3
  Prismatic1 : mblibv1/Joints/Prismatic  LConnTagsString=__newl0|SA1  RConnTagsString=__newr0  UpdateFromCAD=off  NumSAPorts=1  CutJoint=off  MarkAsCut=off  Primitives=prismatic  PrimitiveProps=P1$World$[0 1 0]$prismatic  DialogClass=JointBlock  P1Axis=[0 1 0]
  Scope1 : Scope
      settings: SaveName=force_L
  Scope3 : Scope
      settings: SaveName=toe_position_L
  Selector1 : Selector  InputPortWidth=3  IndexOptions=Index vector (dialog)  Indices=[2]  OutputSizes=1
  Selector2 : Selector  InputPortWidth=3  IndexOptions=Index vector (dialog)  Indices=[2]  OutputSizes=1
  Sine Wave : Sin  Amplitude=waveAmp  Frequency=waveFreq  Phase=wphase  SampleTime=0
  Subsystem : Subsystem
  Sum : Sum  Inputs=++|
  Transport Delay : TransportDelay  DelayTime=5
  Conn1 : PMIOPort  Port=1  Side=Left
  toe_pos : Outport
  wires:
  Body Sensor1/2 -> Selector2/1
  Selector1/1 -> Sum/2, Scope3/1, toe_pos/1  "toe pos"
  Selector2/1 -> Subsystem/2(vel)
  Subsystem/1(force) -> Scope1/1, Mux1/2  "force"
  Mux1/1 -> Body Actuator/1
  Constant/1 -> Mux1/1, Mux1/3
  PVA/1 -> Joint Actuator/1
  Body Sensor1/1 -> Selector1/1
  Sine Wave/1 -> Transport Delay/1
  Sum/1 -> Subsystem/1(pos)
  Transport Delay/1 -> Sum/1
  connections:
  Body1/LConn1 -- Prismatic1/RConn1
  Body Actuator/RConn1 -- Body1/RConn1
  Body Sensor1/LConn1 -- Body1/RConn2
  Prismatic1/LConn1 -- Conn1/RConn1
  Joint Actuator/RConn1 -- Prismatic1/LConn2

== system water_4hopper_open/CPG_Network2/FL_HL lag ==
  In1 : Inport
  In2 : Inport  Port=2
  Constant : Constant  Value=d_phase
  Gain : Gain  Gain=-1
  Sum : Sum  Inputs=--+
  sin : Fcn  Expr=coupling_weight*sin(u(1))
  Out1 : Outport
  Out2 : Outport  Port=2
  wires:
  Sum/1 -> sin/1
  sin/1 -> Gain/1, Out1/1
  Constant/1 -> Sum/2
  In1/1 -> Sum/1
  In2/1 -> Sum/3
  Gain/1 -> Out2/1

== system water_4hopper_open/CPG_Network2/FR_FL lag ==
  In1 : Inport
  In2 : Inport  Port=2
  Constant : Constant  Value=d_phase
  Gain : Gain  Gain=-1
  Sum : Sum  Inputs=--+
  sin : Fcn  Expr=coupling_weight*sin(u(1))
  Out1 : Outport
  Out2 : Outport  Port=2
  wires:
  Sum/1 -> sin/1
  sin/1 -> Gain/1, Out1/1
  Constant/1 -> Sum/2
  In1/1 -> Sum/1
  In2/1 -> Sum/3
  Gain/1 -> Out2/1

== system water_4hopper_open/CPG_Network2/FR_HR lag ==
  In1 : Inport
  In2 : Inport  Port=2
  Constant : Constant  Value=d_phase
  Gain : Gain  Gain=-1
  Sum : Sum  Inputs=--+
  sin : Fcn  Expr=coupling_weight*sin(u(1))
  Out1 : Outport
  Out2 : Outport  Port=2
  wires:
  Gain/1 -> Out2/1
  In2/1 -> Sum/3
  In1/1 -> Sum/1
  Constant/1 -> Sum/2
  sin/1 -> Out1/1, Gain/1
  Sum/1 -> sin/1

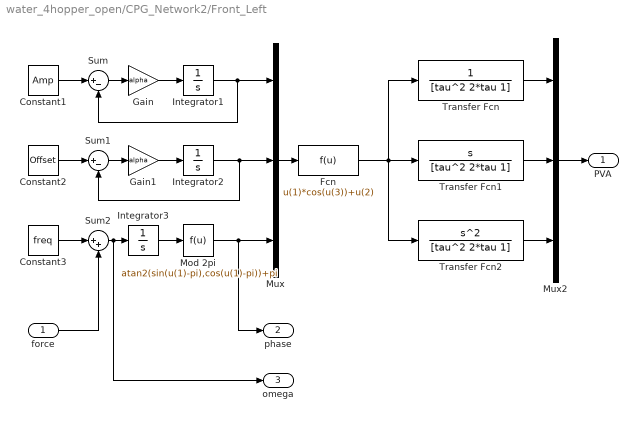
== system water_4hopper_open/CPG_Network2/Front_Left ==
  force : Inport
  Constant1 : Constant  Value=Amp
  Constant2 : Constant  Value=Offset
  Constant3 : Constant  Value=freq
  Fcn : Fcn  Expr=u(1)*cos(u(3))+u(2)
  Gain : Gain  Gain=alpha
  Gain1 : Gain  Gain=alpha
  Integrator1 : Integrator
  Integrator2 : Integrator
  Integrator3 : Integrator  InitialCondition=init_phi + 0.01*rand
  Mod 2pi : Fcn  Expr=atan2(sin(u(1)-pi),cos(u(1)-pi))+pi
  Mux : Mux  Inputs=3
  Mux2 : Mux  Inputs=3
  Sum : Sum  Inputs=|+-
  Sum1 : Sum  Inputs=|+-
  Sum2 : Sum  Inputs=|++
  Transfer Fcn : TransferFcn  Denominator=[tau^2 2*tau 1]
  Transfer Fcn1 : TransferFcn  Numerator=[1 0]  Denominator=[tau^2 2*tau 1]
  Transfer Fcn2 : TransferFcn  Numerator=[1 0 0]  Denominator=[tau^2 2*tau 1]
  PVA : Outport
  phase : Outport  Port=2
  omega : Outport  Port=3
  wires:
  Sum/1 -> Gain/1
  Integrator1/1 -> Sum/2, Mux/1
  Constant1/1 -> Sum/1
  Gain/1 -> Integrator1/1
  Sum1/1 -> Gain1/1
  Integrator2/1 -> Sum1/2, Mux/2
  Constant2/1 -> Sum1/1
  Gain1/1 -> Integrator2/1
  Mux/1 -> Fcn/1
  Mod 2pi/1 -> phase/1, Mux/3
  Integrator3/1 -> Mod 2pi/1
  Constant3/1 -> Sum2/1
  Sum2/1 -> omega/1, Integrator3/1
  force/1 -> Sum2/2
  Transfer Fcn2/1 -> Mux2/3
  Transfer Fcn/1 -> Mux2/1
  Transfer Fcn1/1 -> Mux2/2
  Fcn/1 -> Transfer Fcn2/1, Transfer Fcn/1, Transfer Fcn1/1
  Mux2/1 -> PVA/1

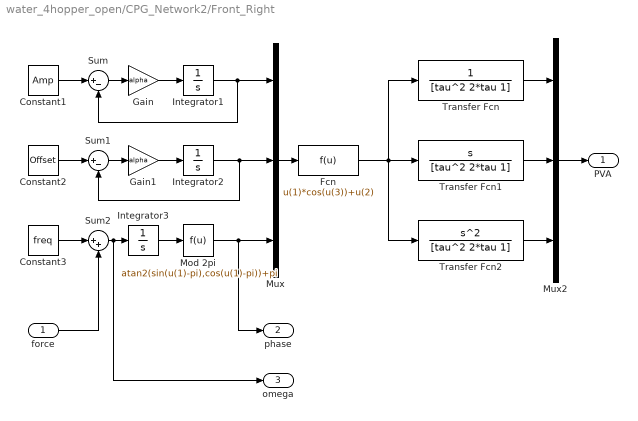
== system water_4hopper_open/CPG_Network2/Front_Right ==
  force : Inport
  Constant1 : Constant  Value=Amp
  Constant2 : Constant  Value=Offset
  Constant3 : Constant  Value=freq
  Fcn : Fcn  Expr=u(1)*cos(u(3))+u(2)
  Gain : Gain  Gain=alpha
  Gain1 : Gain  Gain=alpha
  Integrator1 : Integrator
  Integrator2 : Integrator
  Integrator3 : Integrator  InitialCondition=init_phi + 0.01*rand
  Mod 2pi : Fcn  Expr=atan2(sin(u(1)-pi),cos(u(1)-pi))+pi
  Mux : Mux  Inputs=3
  Mux2 : Mux  Inputs=3
  Sum : Sum  Inputs=|+-
  Sum1 : Sum  Inputs=|+-
  Sum2 : Sum  Inputs=|++
  Transfer Fcn : TransferFcn  Denominator=[tau^2 2*tau 1]
  Transfer Fcn1 : TransferFcn  Numerator=[1 0]  Denominator=[tau^2 2*tau 1]
  Transfer Fcn2 : TransferFcn  Numerator=[1 0 0]  Denominator=[tau^2 2*tau 1]
  PVA : Outport
  phase : Outport  Port=2
  omega : Outport  Port=3
  wires:
  Sum/1 -> Gain/1
  Integrator1/1 -> Sum/2, Mux/1
  Constant1/1 -> Sum/1
  Gain/1 -> Integrator1/1
  Sum1/1 -> Gain1/1
  Integrator2/1 -> Sum1/2, Mux/2
  Constant2/1 -> Sum1/1
  Gain1/1 -> Integrator2/1
  Mux/1 -> Fcn/1
  Mod 2pi/1 -> phase/1, Mux/3
  Integrator3/1 -> Mod 2pi/1
  Constant3/1 -> Sum2/1
  Sum2/1 -> omega/1, Integrator3/1
  force/1 -> Sum2/2
  Transfer Fcn2/1 -> Mux2/3
  Transfer Fcn/1 -> Mux2/1
  Transfer Fcn1/1 -> Mux2/2
  Fcn/1 -> Transfer Fcn2/1, Transfer Fcn/1, Transfer Fcn1/1
  Mux2/1 -> PVA/1

== system water_4hopper_open/CPG_Network2/HR_HL lag ==
  In1 : Inport
  In2 : Inport  Port=2
  Constant : Constant  Value=d_phase
  Gain : Gain  Gain=-1
  Sum : Sum  Inputs=--+
  sin : Fcn  Expr=coupling_weight*sin(u(1))
  Out1 : Outport
  Out2 : Outport  Port=2
  wires:
  Gain/1 -> Out2/1
  In2/1 -> Sum/3
  In1/1 -> Sum/1
  Constant/1 -> Sum/2
  sin/1 -> Out1/1, Gain/1
  Sum/1 -> sin/1

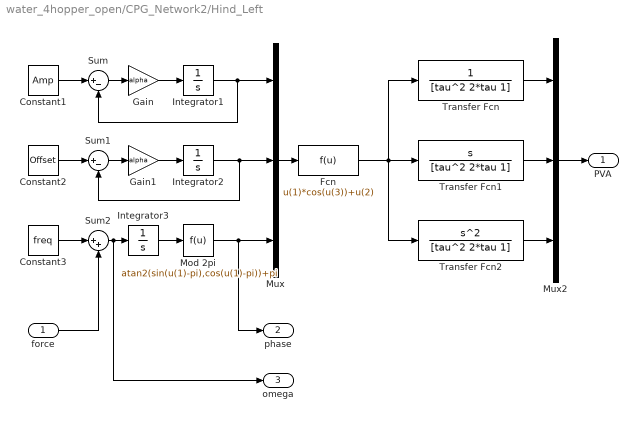
== system water_4hopper_open/CPG_Network2/Hind_Left ==
  force : Inport
  Constant1 : Constant  Value=Amp
  Constant2 : Constant  Value=Offset
  Constant3 : Constant  Value=freq
  Fcn : Fcn  Expr=u(1)*cos(u(3))+u(2)
  Gain : Gain  Gain=alpha
  Gain1 : Gain  Gain=alpha
  Integrator1 : Integrator
  Integrator2 : Integrator
  Integrator3 : Integrator  InitialCondition=init_phi + 0.01*rand
  Mod 2pi : Fcn  Expr=atan2(sin(u(1)-pi),cos(u(1)-pi))+pi
  Mux : Mux  Inputs=3
  Mux2 : Mux  Inputs=3
  Sum : Sum  Inputs=|+-
  Sum1 : Sum  Inputs=|+-
  Sum2 : Sum  Inputs=|++
  Transfer Fcn : TransferFcn  Denominator=[tau^2 2*tau 1]
  Transfer Fcn1 : TransferFcn  Numerator=[1 0]  Denominator=[tau^2 2*tau 1]
  Transfer Fcn2 : TransferFcn  Numerator=[1 0 0]  Denominator=[tau^2 2*tau 1]
  PVA : Outport
  phase : Outport  Port=2
  omega : Outport  Port=3
  wires:
  Sum/1 -> Gain/1
  Integrator1/1 -> Sum/2, Mux/1
  Constant1/1 -> Sum/1
  Gain/1 -> Integrator1/1
  Sum1/1 -> Gain1/1
  Integrator2/1 -> Sum1/2, Mux/2
  Constant2/1 -> Sum1/1
  Gain1/1 -> Integrator2/1
  Mux/1 -> Fcn/1
  Mod 2pi/1 -> phase/1, Mux/3
  Integrator3/1 -> Mod 2pi/1
  Constant3/1 -> Sum2/1
  Sum2/1 -> omega/1, Integrator3/1
  force/1 -> Sum2/2
  Transfer Fcn2/1 -> Mux2/3
  Transfer Fcn/1 -> Mux2/1
  Transfer Fcn1/1 -> Mux2/2
  Fcn/1 -> Transfer Fcn2/1, Transfer Fcn/1, Transfer Fcn1/1
  Mux2/1 -> PVA/1

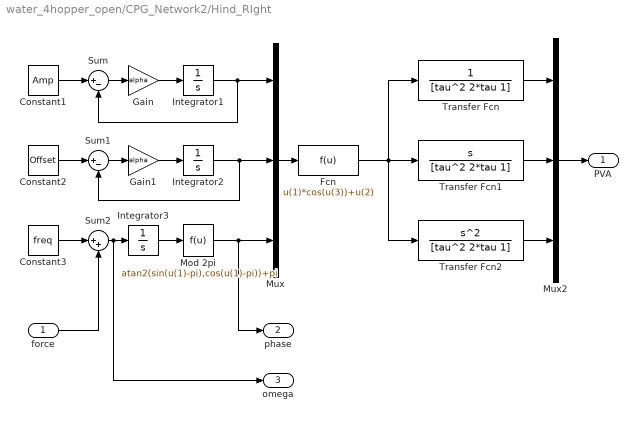
== system water_4hopper_open/CPG_Network2/Hind_RIght ==
  force : Inport
  Constant1 : Constant  Value=Amp
  Constant2 : Constant  Value=Offset
  Constant3 : Constant  Value=freq
  Fcn : Fcn  Expr=u(1)*cos(u(3))+u(2)
  Gain : Gain  Gain=alpha
  Gain1 : Gain  Gain=alpha
  Integrator1 : Integrator
  Integrator2 : Integrator
  Integrator3 : Integrator  InitialCondition=init_phi + 0.01*rand
  Mod 2pi : Fcn  Expr=atan2(sin(u(1)-pi),cos(u(1)-pi))+pi
  Mux : Mux  Inputs=3
  Mux2 : Mux  Inputs=3
  Sum : Sum  Inputs=|+-
  Sum1 : Sum  Inputs=|+-
  Sum2 : Sum  Inputs=|++
  Transfer Fcn : TransferFcn  Denominator=[tau^2 2*tau 1]
  Transfer Fcn1 : TransferFcn  Numerator=[1 0]  Denominator=[tau^2 2*tau 1]
  Transfer Fcn2 : TransferFcn  Numerator=[1 0 0]  Denominator=[tau^2 2*tau 1]
  PVA : Outport
  phase : Outport  Port=2
  omega : Outport  Port=3
  wires:
  Sum/1 -> Gain/1
  Integrator1/1 -> Sum/2, Mux/1
  Constant1/1 -> Sum/1
  Gain/1 -> Integrator1/1
  Sum1/1 -> Gain1/1
  Integrator2/1 -> Sum1/2, Mux/2
  Constant2/1 -> Sum1/1
  Gain1/1 -> Integrator2/1
  Mux/1 -> Fcn/1
  Mod 2pi/1 -> phase/1, Mux/3
  Integrator3/1 -> Mod 2pi/1
  Constant3/1 -> Sum2/1
  Sum2/1 -> omega/1, Integrator3/1
  force/1 -> Sum2/2
  Transfer Fcn2/1 -> Mux2/3
  Transfer Fcn/1 -> Mux2/1
  Transfer Fcn1/1 -> Mux2/2
  Fcn/1 -> Transfer Fcn2/1, Transfer Fcn/1, Transfer Fcn1/1
  Mux2/1 -> PVA/1

== system water_4hopper_open/CPG_Network2/split FL ==
  w_pos : Inport
  PVA : Inport  Port=2
  w_neg : Inport  Port=3
  Product : Product  RndMeth=Zero
  Product1 : Product  RndMeth=Zero
  Sum2 : Sum  Inputs=|++
  enable : Subsystem
  sel : Selector  InputPortWidth=3  IndexOptions=Index vector (dialog)  Indices=[2]  OutputSizes=1
  Force : Outport
  wires:
  Product/1 -> Sum2/1
  w_pos/1 -> Product/1
  w_neg/1 -> Product1/1
  Product1/1 -> Sum2/2
  PVA/1 -> sel/1
  enable/1(pos) -> Product/2
  enable/2(neg) -> Product1/2
  Sum2/1 -> Force/1
  sel/1 -> enable/1(in)

== system water_4hopper_open/CPG_Network2/split FL1 ==
  w_pos : Inport
  PVA : Inport  Port=2
  w_neg : Inport  Port=3
  Product : Product  RndMeth=Zero
  Product1 : Product  RndMeth=Zero
  Sum2 : Sum  Inputs=|++
  enable : Subsystem
  sel : Selector  InputPortWidth=3  IndexOptions=Index vector (dialog)  Indices=[2]  OutputSizes=1
  Force : Outport
  wires:
  sel/1 -> enable/1(in)
  Sum2/1 -> Force/1
  enable/2(neg) -> Product1/2
  enable/1(pos) -> Product/2
  PVA/1 -> sel/1
  Product1/1 -> Sum2/2
  w_neg/1 -> Product1/1
  w_pos/1 -> Product/1
  Product/1 -> Sum2/1

== system water_4hopper_open/CPG_Network2/split FL2 ==
  w_pos : Inport
  PVA : Inport  Port=2
  w_neg : Inport  Port=3
  Product : Product  RndMeth=Zero
  Product1 : Product  RndMeth=Zero
  Sum2 : Sum  Inputs=|++
  enable : Subsystem
  sel : Selector  InputPortWidth=3  IndexOptions=Index vector (dialog)  Indices=[2]  OutputSizes=1
  Force : Outport
  wires:
  Product/1 -> Sum2/1
  w_pos/1 -> Product/1
  w_neg/1 -> Product1/1
  Product1/1 -> Sum2/2
  PVA/1 -> sel/1
  enable/1(pos) -> Product/2
  enable/2(neg) -> Product1/2
  Sum2/1 -> Force/1
  sel/1 -> enable/1(in)

== system water_4hopper_open/CPG_Network2/split FL3 ==
  w_pos : Inport
  PVA : Inport  Port=2
  w_neg : Inport  Port=3
  Product : Product  RndMeth=Zero
  Product1 : Product  RndMeth=Zero
  Sum2 : Sum  Inputs=|++
  enable : Subsystem
  sel : Selector  InputPortWidth=3  IndexOptions=Index vector (dialog)  Indices=[2]  OutputSizes=1
  Force : Outport
  wires:
  Product/1 -> Sum2/1
  w_pos/1 -> Product/1
  w_neg/1 -> Product1/1
  Product1/1 -> Sum2/2
  PVA/1 -> sel/1
  enable/1(pos) -> Product/2
  enable/2(neg) -> Product1/2
  Sum2/1 -> Force/1
  sel/1 -> enable/1(in)

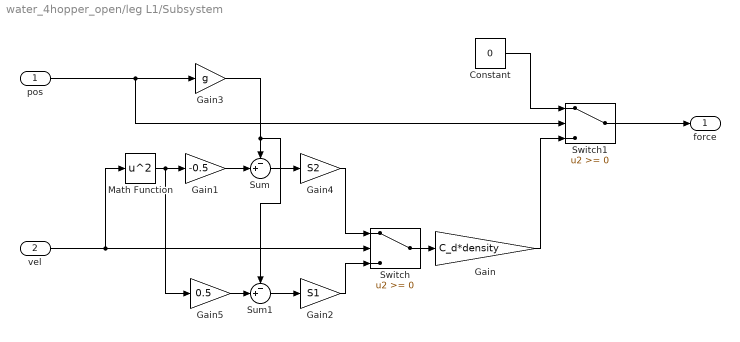
== system water_4hopper_open/leg L1/Subsystem ==
  pos : Inport
  vel : Inport  Port=2
  Constant : Constant  Value=0
  Gain : Gain  Gain=C_d*density
  Gain1 : Gain  Gain=-0.5
  Gain2 : Gain  Gain=S1
  Gain3 : Gain  Gain=g
  Gain4 : Gain  Gain=S2
  Gain5 : Gain  Gain=0.5
  Math Function : Math  Operator=square  SaturateOnIntegerOverflow=on
  Sum : Sum  Inputs=-+|
  Sum1 : Sum  Inputs=-+|
  Switch : Switch  ZeroCross=off
  Switch1 : Switch
  force : Outport
  wires:
  vel/1 -> Switch/2, Math Function/1
  Math Function/1 -> Gain1/1, Gain5/1
  Gain1/1 -> Sum/2
  pos/1 -> Gain3/1, Switch1/2
  Gain3/1 -> Sum/1, Sum1/1
  Sum/1 -> Gain4/1
  Gain4/1 -> Switch/1
  Gain2/1 -> Switch/3
  Switch/1 -> Gain/1
  Switch1/1 -> force/1
  Gain/1 -> Switch1/3
  Constant/1 -> Switch1/1
  Sum1/1 -> Gain2/1
  Gain5/1 -> Sum1/2

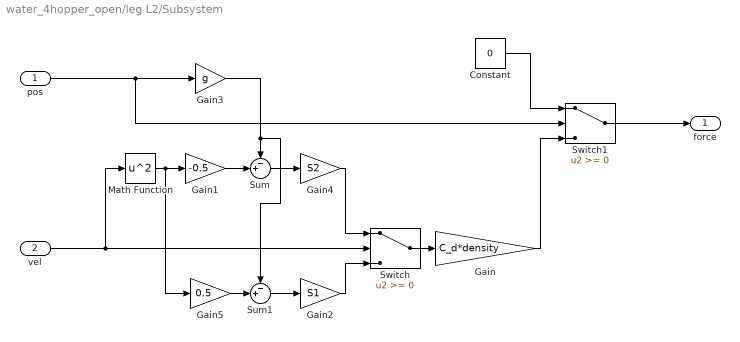
== system water_4hopper_open/leg L2/Subsystem ==
  pos : Inport
  vel : Inport  Port=2
  Constant : Constant  Value=0
  Gain : Gain  Gain=C_d*density
  Gain1 : Gain  Gain=-0.5
  Gain2 : Gain  Gain=S1
  Gain3 : Gain  Gain=g
  Gain4 : Gain  Gain=S2
  Gain5 : Gain  Gain=0.5
  Math Function : Math  Operator=square  SaturateOnIntegerOverflow=on
  Sum : Sum  Inputs=-+|
  Sum1 : Sum  Inputs=-+|
  Switch : Switch  ZeroCross=off
  Switch1 : Switch
  force : Outport
  wires:
  vel/1 -> Switch/2, Math Function/1
  Math Function/1 -> Gain1/1, Gain5/1
  Gain1/1 -> Sum/2
  pos/1 -> Gain3/1, Switch1/2
  Gain3/1 -> Sum/1, Sum1/1
  Sum/1 -> Gain4/1
  Gain4/1 -> Switch/1
  Gain2/1 -> Switch/3
  Switch/1 -> Gain/1
  Switch1/1 -> force/1
  Gain/1 -> Switch1/3
  Constant/1 -> Switch1/1
  Sum1/1 -> Gain2/1
  Gain5/1 -> Sum1/2

== system water_4hopper_open/leg L3/Subsystem ==
  pos : Inport
  vel : Inport  Port=2
  Constant : Constant  Value=0
  Gain : Gain  Gain=C_d*density
  Gain1 : Gain  Gain=-0.5
  Gain2 : Gain  Gain=S1
  Gain3 : Gain  Gain=g
  Gain4 : Gain  Gain=S2
  Gain5 : Gain  Gain=0.5
  Math Function : Math  Operator=square  SaturateOnIntegerOverflow=on
  Sum : Sum  Inputs=-+|
  Sum1 : Sum  Inputs=-+|
  Switch : Switch  ZeroCross=off
  Switch1 : Switch
  force : Outport
  wires:
  vel/1 -> Switch/2, Math Function/1
  Math Function/1 -> Gain1/1, Gain5/1
  Gain1/1 -> Sum/2
  pos/1 -> Gain3/1, Switch1/2
  Gain3/1 -> Sum/1, Sum1/1
  Sum/1 -> Gain4/1
  Gain4/1 -> Switch/1
  Gain2/1 -> Switch/3
  Switch/1 -> Gain/1
  Switch1/1 -> force/1
  Gain/1 -> Switch1/3
  Constant/1 -> Switch1/1
  Sum1/1 -> Gain2/1
  Gain5/1 -> Sum1/2

== system water_4hopper_open/leg L4/Subsystem ==
  pos : Inport
  vel : Inport  Port=2
  Constant : Constant  Value=0
  Gain : Gain  Gain=C_d*density
  Gain1 : Gain  Gain=-0.5
  Gain2 : Gain  Gain=S1
  Gain3 : Gain  Gain=g
  Gain4 : Gain  Gain=S2
  Gain5 : Gain  Gain=0.5
  Math Function : Math  Operator=square  SaturateOnIntegerOverflow=on
  Sum : Sum  Inputs=-+|
  Sum1 : Sum  Inputs=-+|
  Switch : Switch  ZeroCross=off
  Switch1 : Switch
  force : Outport
  wires:
  vel/1 -> Switch/2, Math Function/1
  Math Function/1 -> Gain1/1, Gain5/1
  Gain1/1 -> Sum/2
  pos/1 -> Gain3/1, Switch1/2
  Gain3/1 -> Sum/1, Sum1/1
  Sum/1 -> Gain4/1
  Gain4/1 -> Switch/1
  Gain2/1 -> Switch/3
  Switch/1 -> Gain/1
  Switch1/1 -> force/1
  Gain/1 -> Switch1/3
  Constant/1 -> Switch1/1
  Sum1/1 -> Gain2/1
  Gain5/1 -> Sum1/2

== system water_4hopper_open/CPG_Network2/split FL/enable ==
  in : Inport
  Constant1 : Constant
  Constant2 : Constant
  Derivative : Derivative
  Gain : Gain  Gain=.5
  Gain1 : Gain  Gain=.5
  Sign : Signum
  Sum1 : Sum  Inputs=|++
  Sum2 : Sum  Inputs=|-+
  pos : Outport
  neg : Outport  Port=2
  wires:
  Derivative/1 -> Sign/1
  Constant1/1 -> Sum1/2
  Sign/1 -> Sum2/1, Sum1/1
  Gain/1 -> pos/1
  in/1 -> Derivative/1
  Sum1/1 -> Gain/1
  Constant2/1 -> Sum2/2
  Gain1/1 -> neg/1
  Sum2/1 -> Gain1/1

== system water_4hopper_open/CPG_Network2/split FL1/enable ==
  in : Inport
  Constant1 : Constant
  Constant2 : Constant
  Derivative : Derivative
  Gain : Gain  Gain=.5
  Gain1 : Gain  Gain=.5
  Sign : Signum
  Sum1 : Sum  Inputs=|++
  Sum2 : Sum  Inputs=|-+
  pos : Outport
  neg : Outport  Port=2
  wires:
  Sum2/1 -> Gain1/1
  Gain1/1 -> neg/1
  Constant2/1 -> Sum2/2
  Sum1/1 -> Gain/1
  in/1 -> Derivative/1
  Gain/1 -> pos/1
  Sign/1 -> Sum1/1, Sum2/1
  Constant1/1 -> Sum1/2
  Derivative/1 -> Sign/1

== system water_4hopper_open/CPG_Network2/split FL2/enable ==
  in : Inport
  Constant1 : Constant
  Constant2 : Constant
  Derivative : Derivative
  Gain : Gain  Gain=.5
  Gain1 : Gain  Gain=.5
  Sign : Signum
  Sum1 : Sum  Inputs=|++
  Sum2 : Sum  Inputs=|-+
  pos : Outport
  neg : Outport  Port=2
  wires:
  Derivative/1 -> Sign/1
  Constant1/1 -> Sum1/2
  Sign/1 -> Sum2/1, Sum1/1
  Gain/1 -> pos/1
  in/1 -> Derivative/1
  Sum1/1 -> Gain/1
  Constant2/1 -> Sum2/2
  Gain1/1 -> neg/1
  Sum2/1 -> Gain1/1
